simulink model "Simulation_wrapped_4"  (R2015a)
settings: Solver=ode4  SolverMode=SingleTasking  StartTime=0.0  StopTime=20  FixedStep=0.001  MaxStep=0.01  RelTol=1e-3
InitFcn:
  | gen_signal
  | Read_aero_spreadsheet
  | model_params3
undefined symbols (not defined in the file or in its folder): acm_aero_model, acm_pitch_deg_ini, acm_pitch_rate_deg_s_ini, acm_T_N, breakpoints1, Cm0, Cmde, Cmq, dail, de, dele, drud, Fr_mp_1, Fr_mp_2, Fr_rp_1, Fr_rp_2, ini_acm_de_deg, ini_acm_p_deg_per_s, ini_acm_phi_deg, ini_acm_psi_deg, ini_acm_q_deg_per_s, ini_acm_r_deg_per_s, ini_acm_theta_deg, ini_cmp_de_deg, ini_rig_p_deg_per_s, ini_rig_phi_deg, ini_rig_psi_deg, ini_rig_q_deg_per_s, ini_rig_r_deg_per_s, ini_rig_theta_deg, ini_rig_theta_deg_per_s, K1_svo_acm, K1_svo_cmp, K2_svo_acm, K2_svo_cmp, K_de_nz2, K_de_q2, K_de_tht2, La, Ma, max_defl_sat_acm, max_defl_sat_cmp, max_rate_sat, max_rate_sat_acm, max_rate_sat_cmp, Na, rig_pitch_deg_ini, rig_pitch_rate_deg_s_ini, sigbuilder_block, simstop, windspeed, Xa, Ya, Za
libraries: aerolibconvert2 x96, simulink x40, aerolibtransform2 x18, vrlib x7
(part 2 of 6)

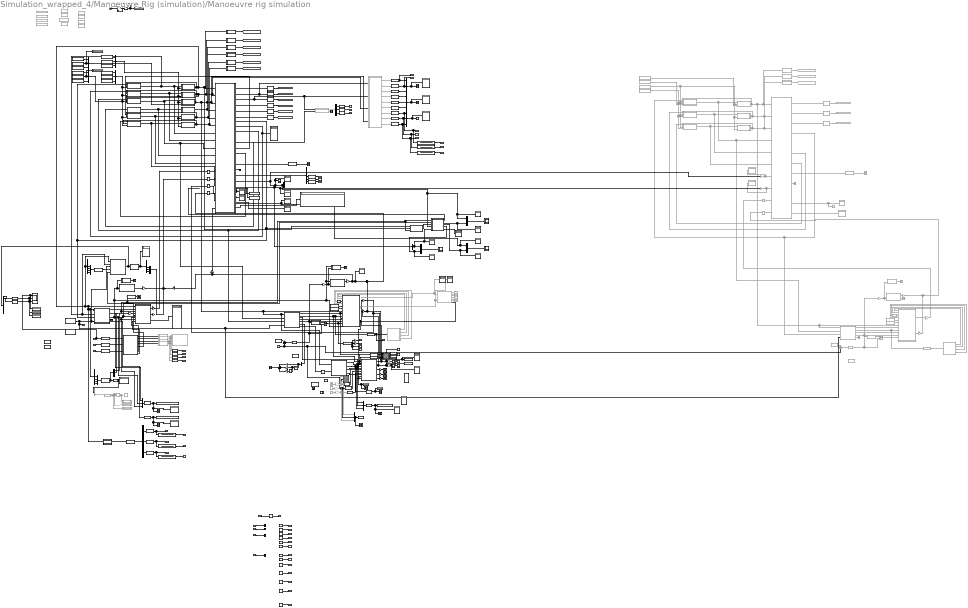
== system Simulation_wrapped_4/Manoeuvre Rig (simulation)/Manoeuvre rig simulation ==
  note: yaw
  note: pitch
  note: roll
  note: Estimated reaction forces
  note: Simulation aircraft reaction forces
  note: Estimated laod cell reading
  note: Simulation load cell reading
  note: ALTITUDE CONTROL
  note: Estimated estimated load cell moment
  note: Simulation load cell moment
  clock : Inport
  ACM_da_c(deg) : Inport  Port=2
  ACM_dea_c(deg) : Inport  Port=3
  ACM_de_c(deg) : Inport  Port=4
  ACM_dr_c(deg) : Inport  Port=5
  CMP_da_c(deg) : Inport  Port=6
  CMP_de_c(deg) : Inport  Port=7
  CMP_dr_c(deg) : Inport  Port=8
  extra : Inport  Port=9
  Aerodynamics lookup : Subsystem  Commented=on
  Aerodynamics lookup1 : Subsystem  Commented=on
  Aerodynamics model: Hawk : MATLAB Function
      settings: MinAlgLoopOccurrences=on
  Aerodynamics model: Hawk1 : MATLAB Function  Commented=on
      settings: MinAlgLoopOccurrences=on
  Aerodynamics model: compensator : MATLAB Function
      settings: MinAlgLoopOccurrences=on
  Aileron command (differential) : Terminator
  Aircraft acceleration body axis : MATLAB Function  Commented=on  TreatAsAtomicUnit=on
  Aircraft attitude relative to arm2 : MATLAB Function  Commented=on  TreatAsAtomicUnit=on
  Aircraft loads for load case loop : MATLAB Function  Commented=on
      settings: MinAlgLoopOccurrences=on
  Aircraft model vertical reaction force : Scope
      settings: YMin=5  YMax=24  SaveName=ScopeData38
  Aircraft model vertical reaction force1 : Scope  Commented=on
      settings: YMin=5  YMax=24
  Aircraft_model_friction : MATLAB Function
      settings: MinAlgLoopOccurrences=on
  Aircraft_model_friction1 : MATLAB Function  Commented=on
      settings: MinAlgLoopOccurrences=on
  Angle Conversion{,1,3,6,8..12,14..26,29..34,37..38,40} (31 alike) : aerolibconvert2/Angle Conversion  IU=rad  OU=deg
  Angle Conversion{2,4,7,13,27..28,35,39} (8 alike) : aerolibconvert2/Angle Conversion  IU=deg  OU=rad
  Angle Conversion36 : aerolibconvert2/Angle Conversion  Commented=on  IU=deg  OU=rad
  Angle Conversion44 : aerolibconvert2/Angle Conversion  Commented=on  IU=deg  OU=rad
  Angle Conversion5 : aerolibconvert2/Angle Conversion  Commented=on  IU=rad  OU=deg
  Angle of sideslip : Constant  Value=0
  Butterworth filter (cutoff frequency 10Hz) + differentiating{,1..5} (6 alike) : TransferFcn  Numerator=[1 0]  Denominator=[2.5330e-04 0.0225 1]
  CMP aero model : MATLABFcn  MATLABFcn=Cmp_aero_model
  Calculating rig pitch acceleration : MATLAB Function  TreatAsAtomicUnit=on
  Chirp Signal : simulink/Sources/Chirp Signal  Commented=on  f1=0.5  T=120  f2=3
  Chirp Signal1 : simulink/Sources/Chirp Signal  Commented=on  f1=0.5  T=120  f2=3
  Chirp Signal2 : simulink/Sources/Chirp Signal  f1=0.5  T=120  f2=3
  Clock : Clock
  Comparing simulation aircraft reaction forces and estimated reaction forces : Scope
      settings: YMin=-35  YMax=15  SaveName=ScopeData3
  Comparing simulation aircraft reaction forces and estimated reaction forces1 : Scope
      settings: YMin=-35  YMax=15  SaveName=ScopeData4
  Comparing simulation load cell reading and estimated load cell reading : Scope
      settings: YMin=-17.5  YMax=37.5  SaveName=ScopeData2
  Compensator friction : MATLAB Function
      settings: MinAlgLoopOccurrences=on
  Compensator servo model1 : Subsystem  Commented=on
  Compensator servo model2 : Subsystem  Commented=on
  Compensator servo model3 : Subsystem  Commented=on
  Compensator servo model4 : Subsystem  Commented=on
  Constant : Constant  Commented=on  Value=simstop
  Constant{1,7..8,12..13,19} (6 alike) : Constant  Commented=on  Value=0
  Constant10 : Constant  Value=7.515637662
  Constant11 : Constant  Value=0
  Constant14 : Constant  Commented=on  Value=2.6111
  Constant15 : Constant  Commented=on  Value=rig_pitch_rate_deg_s_ini
  Constant16 : Constant  Commented=on  Value=acm_pitch_rate_deg_s_ini
  Constant17 : Constant  Commented=on  Value=rig_pitch_deg_ini
  Constant18 : Constant  Commented=on  Value=acm_pitch_deg_ini
  Constant2 : Constant  Value=-7.308232274
  Constant3 : Constant  Value=14.34612797
  Constant4 : Constant  Commented=on  Value=-7.308232274
  Constant6 : Constant  Commented=on  Value=5
  Cq_transpose_lc CHECK : Display
  Demux : Demux  Outputs=7
  Demux{1..3,5..6,12} (6 alike) : Demux  Outputs=3
  Demux10 : Demux  Outputs=11
  Demux4 : Demux  Commented=on  Outputs=3
  Demux7 : Demux  Outputs=6
  Demux8 : Demux  Outputs=7
  Demux9 : Demux  Outputs=6
  Derivative : Derivative
  Display{,2..3,5..14,18} (14 alike) : Display
  Display{1,4,15..17} (5 alike) : Display  Commented=on
  Elevator command (differential) : Terminator
  Equations of Motion : MATLAB Function
      settings: MinAlgLoopOccurrences=on
  Equations of Motion1 : MATLAB Function  Commented=on
      settings: MinAlgLoopOccurrences=on
  Extra : Terminator
  Extracting aircraft vertical reaction forces1 : MATLAB Function  TreatAsAtomicUnit=on
  Extracting aircraft vertical reaction forces2 : MATLAB Function  Commented=on  TreatAsAtomicUnit=on
  Extracting position vector 1 : Subsystem
  Extracting position vector 10 : Subsystem  Commented=on
  Extracting position vector 2 : Subsystem
  "Extracting position vector 2 " : Subsystem
  Extracting position vector 3 : Subsystem
  Extracting position vector 4 : Subsystem
  Extracting position vector 5 : Subsystem
  Extracting position vector 7 : Subsystem  Commented=on
  Extracting position vector 8 : Subsystem  Commented=on
  F : Display
  FF : Display
  Fcn : Fcn  Expr=u/9.81
  Fcn1 : Fcn  Expr=u/9.81
  Fcn2 : Fcn  Expr=u/9.81
  Friction_estimate : Display
  Friction_moment : Display
  Gain{,3,6..7,11,14,28} (7 alike) : Gain  Gain=-1
  Gain1 : Gain  Commented=on  Gain=-1
  Gain{4,8..10,17,19..23,30} (11 alike) : Gain
  Gain12 : Gain  Gain=0
  Gain13 : Gain  Gain=0
  Gain15 : Gain  Commented=on  Gain=-1
  Gain16 : Gain  Commented=on  Gain=0
  Gain18 : Gain  Commented=on
  Gain2 : Gain  Commented=on
  Gain24 : Gain  Commented=on  Gain=dail
  Gain25 : Gain  Commented=on  Gain=dele
  Gain26 : Gain  Commented=on
  Gain27 : Gain  Commented=on  Gain=drud
  Goto10 : Goto  Commented=on  GotoTag=animation_l2_translation  TagVisibility=global
  Goto15 : Goto  Commented=on  GotoTag=animation_acm2_rotation  TagVisibility=global
  Goto16 : Goto  Commented=on  GotoTag=animation_lc2_rotation  TagVisibility=global
  Goto17 : Goto  Commented=on  GotoTag=animation_l2_rotation  TagVisibility=global
  Goto8 : Goto  Commented=on  GotoTag=animation_acm2_translation  TagVisibility=global
  Goto9 : Goto  Commented=on  GotoTag=animation_lc2_translation  TagVisibility=global
  HHIRM : MATLAB Function
      settings: MinAlgLoopOccurrences=on
  Hawk servo model : Subsystem
  Hawk servo model1 : Subsystem  Commented=on
  IC{1..4} (4 alike) : InitialCondition  Value=0
  IC7 : InitialCondition  Commented=on  Value=0
  IC8 : InitialCondition  Commented=on  Value=0
  Integrator : Integrator
  Integrator1 : Integrator
  L : Constant  Commented=on  Value=La
  Left aileron command : Constant  Value=0
  Left aileron measured : Constant  Value=0
  Load cell reading to aircraft reaction forces : MATLAB Function  TreatAsAtomicUnit=on
  M : Display
  M1 : Constant  Commented=on  Value=Ma
  MATLAB Function1 : MATLAB Function  TreatAsAtomicUnit=on
  MATLAB Function10 : MATLAB Function  TreatAsAtomicUnit=on
  MATLAB Function11 : MATLAB Function  Commented=on  TreatAsAtomicUnit=on
  MATLAB Function13 : MATLAB Function  Commented=on
      settings: MinAlgLoopOccurrences=on
  MATLAB Function15 : MATLAB Function  Commented=on  TreatAsAtomicUnit=on
  MATLAB Function18 : MATLAB Function  Commented=on  TreatAsAtomicUnit=on
  MATLAB Function2 : MATLAB Function  TreatAsAtomicUnit=on
  MATLAB Function3 : MATLAB Function
      settings: MinAlgLoopOccurrences=on
  MATLAB Function4 : MATLAB Function  TreatAsAtomicUnit=on
  MATLAB Function5 : MATLAB Function
      settings: MinAlgLoopOccurrences=on
  MATLAB Function6 : MATLAB Function  TreatAsAtomicUnit=on
  MATLAB Function7 : MATLAB Function
      settings: MinAlgLoopOccurrences=on
  MATLAB Function8 : MATLAB Function  TreatAsAtomicUnit=on
  MATLAB Function9 : MATLAB Function  TreatAsAtomicUnit=on
  MM : Display
  Manual Switch1 : ManualSwitch  CurrentSetting=0
  Manual Switch3 : ManualSwitch  Commented=on  CurrentSetting=0
  Memory : Memory
  Mux{,2..4,7..10,12..13,15} (11 alike) : Mux  Inputs=3
  Mux1 : Mux  Inputs=2
  Mux11 : Mux
  Mux14 : Mux
  Mux5 : Mux  Inputs=2
  Mux6 : Mux  Inputs=2
  N : Constant  Commented=on  Value=Na
  Physical deflections to virtual compensator deflections : MATLAB Function  Commented=on  TreatAsAtomicUnit=on
  Quaternions to Rotation Angles : aerolibtransform2/Quaternions to Rotation Angles  rotationOrder=ZYX
  Quaternions to Rotation Angles1 : aerolibtransform2/Quaternions to Rotation Angles  rotationOrder=ZYX
  Quaternions to Rotation Angles2 : aerolibtransform2/Quaternions to Rotation Angles  rotationOrder=ZYX
  Relational Operator : RelationalOperator  Commented=on  OutDataTypeStr=boolean
  Relative angle from rotation matrix : Scope
      settings: ShowLegends=on  YMax=12.5  SaveName=ScopeData17
  Right aileron command : Constant  Value=0
  Right aileron measured : Constant  Value=0
  Rotation angles from rotation matrix (acm) : Scope
      settings: ShowLegends=on  YMax=12.5  SaveName=ScopeData19
  Rotation angles from rotation matrix (arm) : Scope
      settings: ShowLegends=on  YMax=12.5  SaveName=ScopeData20
  Rudder command : Terminator
  Rudder measured : Constant  Value=0
  Rudder measured command : Constant  Value=0
  Scope{,1..8,10..13} (13 alike) : Scope
      Scope settings: YMin=-0.5  YMax=0.2  SaveName=ScopeData6
      Scope1 settings: YMin=0.12  YMax=0.1775  SaveName=ScopeData8
      Scope10 settings: YMin=-3.25  YMax=0  SaveName=ScopeData21
      Scope11 settings: YMin=-17.5  YMax=0  SaveName=ScopeData30
      Scope12 settings: YMin=0  YMax=1000  SaveName=ScopeData33
      Scope13 settings: YMin=-275  YMax=275  SaveName=ScopeData34
      Scope2 settings: YMin=0  YMax=14  SaveName=ScopeData9
      Scope3 settings: YMin=-700  YMax=700  SaveName=ScopeData10
      Scope4 settings: YMin=-8  YMax=8  SaveName=ScopeData11
      Scope5 settings: YMin=-21  YMax=1  SaveName=ScopeData12
      Scope6 settings: YMin=0  YMax=14  SaveName=ScopeData13
      Scope7 settings: YMin=0  YMax=14  SaveName=ScopeData15
      Scope8 settings: YMin=-0.02  YMax=0.0225  SaveName=ScopeData18
  Scope14 : Scope  NumInputPorts=3
      settings: YMin=38~127.5~-1240  YMax=42~157.5~-1190  SaveName=ScopeData35
  Scope9 : TimeScope  NumInputPorts=5
  Signal Builder : Subsystem  Tag=STV Subsys  LoadFcn=sigbuilder_block('load');  StartFcn=sigbuilder_block('start');  StopFcn=sigbuilder_block('stop');  ClipboardFcn=sigbuilder_block('clipboard');  mask(Sigbuilder block){}
      mask help: Simulink:masks:SigbuilderBlock_MD
      mask init:
      | if ~strcmp(get_param(bdroot(gcbh),'SimulationStatus'),'stopped') tuvar = sigbuilder_block('maskInit'); end
      settings: CopyFcn=sigbuilder_block('copy');  DeleteFcn=sigbuilder_block('delete');  ModelCloseFcn=sigbuilder_block('modelClose');  PreSaveFcn=sigbuilder_block('preSave');  PauseFcn=sigbuilder_block('pause');  ContinueFcn=sigbuilder_block('continue');  NameChangeFcn=sigbuilder_block('namechange');  OpenFcn=sigbuilder_block('open',[437.6 199.2 550.4 400 ]);  CloseFcn=sigbuilder_block('close');
      mask Display: plot(0, 0, 100, 100,[2, 2, 32, 32, 2], [68, 8, 8, 68, 68],[32, 2], [38, 38], [32, 19, 2],[53, 60, 44], [32, 17, 17, 2],[16, 16, 31, 31]);txt = getActiveGroup(gcbh);text(2, 100, txt,'verticalAlignment', 'top');
  Step : Step  Commented=on  Time=0.01  SampleTime=0
  Step2 : Step  SampleTime=0
  Step3 : Step  SampleTime=0
  Stop Simulation : Stop  Commented=on
  Subsystem : Subsystem
  Subsystem1 : Subsystem
  Subsystem10 : Subsystem
  Subsystem11 : Subsystem
  Subsystem12 : Subsystem
  Subsystem13 : Subsystem
  Subsystem16 : Subsystem  Commented=on
  Subsystem17 : Subsystem  Commented=on
  Subsystem18 : Subsystem  Commented=on
  Subsystem19 : Subsystem  Commented=on
  Subsystem2 : Subsystem
  Subsystem22 : Subsystem  Commented=on
  Subsystem23 : Subsystem  Commented=on
  Subsystem24 : Subsystem  Commented=on
  Subsystem3 : Subsystem
  Subsystem4 : Subsystem
  Subsystem5 : Subsystem
  Subsystem6 : Subsystem
  Subsystem7 : Subsystem
  Subsystem8 : Subsystem
  Subsystem9 : Subsystem
  Sum1 : Sum  Commented=on  Inputs=|++
  Sum2 : Sum  Inputs=|++
  Sum3 : Sum
  Sum4 : Sum  Commented=on
  Sum5 : Sum  Inputs=+++
  Sum8 : Sum  Inputs=++-
  Switch : Switch  Criteria=u2 > Threshold
  Terminator{,1..5} (6 alike) : Terminator
  Terminator{7..10} (4 alike) : Terminator  Commented=on
  Theta1 : Constant  Commented=on  Value=2.9881840554008
  To Workspace : ToWorkspace  VariableName=reaction_forces_lc_body_N  SaveFormat=Timeseries  SampleTime=-1
  To Workspace1 : ToWorkspace  VariableName=reaction_moments_lc_body_Nm  SaveFormat=Timeseries  SampleTime=-1
  To Workspace2 : ToWorkspace  VariableName=cs_deg  SaveFormat=Timeseries  SampleTime=-1
  To Workspace3 : ToWorkspace  VariableName=alpha_deg  SaveFormat=Timeseries  SampleTime=-1
  To Workspace4 : ToWorkspace  VariableName=beta_deg  SaveFormat=Timeseries  SampleTime=-1
  To Workspace5 : ToWorkspace  VariableName=aero_forces_N  SaveFormat=Timeseries  SampleTime=-1
  To Workspace6 : ToWorkspace  VariableName=aero_moments_Nm  SaveFormat=Timeseries  SampleTime=-1
  To Workspace7 : ToWorkspace  VariableName=wind_axes_rotation_rates_degpers  SaveFormat=Timeseries  SampleTime=-1
  To Workspace8 : ToWorkspace  VariableName=inertial_axes_CMP_rotation_rates_degpers  SaveFormat=Timeseries  SampleTime=-1
  To Workspace9 : ToWorkspace  VariableName=inertial_axes_CMP_rotation_accelerations_degperspers  SaveFormat=Timeseries  SampleTime=-1
  Transport Delay : TransportDelay  DelayTime=0.01
  Unused{,1..2,4,6,8} (6 alike) : Constant  Value=0
  V{,1..3} (4 alike) : Display
  Virtual compensator deflections to physical deflections : MATLAB Function  TreatAsAtomicUnit=on
  Wind axes angular rates calculation : MATLAB Function
      settings: MinAlgLoopOccurrences=on
  Wind tunnel velocity : Constant  Value=windspeed
  Wind tunnel velocity1 : Constant  Value=25.09344509
  X : Constant  Commented=on  Value=Xa
  Y : Constant  Commented=on  Value=Ya
  Z : Constant  Commented=on  Value=Za
  acm_T_N : Constant  Value=acm_T_N
  acm_T_N1 : Constant  Commented=on  Value=acm_T_N
  acm_aero_model : Constant  Value=acm_aero_model
  acm_aero_model1 : Constant  Commented=on  Value=acm_aero_model
  aircraft_cell_reaction_forces : Display
  aircraft_cell_reaction_moments : Display
  alpha : Display
  alpha1 : Display
  alpha2 : Scope
      settings: YMin=-55  YMax=55  SaveName=ScopeData22
  beta2 : Scope
      settings: YMin=-12.25  YMax=-8.75  SaveName=ScopeData23
  ini_acm_q_deg_per_s : Constant  Value=ini_acm_q_deg_per_s
  ini_acm_q_deg_per_s1 : Constant  Commented=on  Value=ini_acm_q_deg_per_s
  ini_acm_q_deg_per_s2 : Constant  Value=ini_acm_p_deg_per_s
  ini_acm_q_deg_per_s3 : Constant  Value=ini_acm_r_deg_per_s
  ini_acm_theta_deg : Constant  Value=ini_acm_theta_deg
  ini_acm_theta_deg1 : Constant  Commented=on  Value=ini_acm_theta_deg
  ini_acm_theta_deg2 : Constant  Value=ini_acm_phi_deg
  ini_acm_theta_deg3 : Constant  Value=ini_acm_psi_deg
  ini_rig_theta_deg : Constant  Value=ini_rig_theta_deg
  ini_rig_theta_deg1 : Constant  Commented=on  Value=ini_rig_theta_deg
  ini_rig_theta_deg2 : Constant  Value=ini_rig_psi_deg
  ini_rig_theta_deg3 : Constant  Value=ini_rig_phi_deg
  ini_rig_theta_deg_per_s : Constant  Value=ini_rig_q_deg_per_s
  ini_rig_theta_deg_per_s1 : Constant  Commented=on  Value=ini_rig_theta_deg_per_s
  ini_rig_theta_deg_per_s2 : Constant  Value=ini_rig_p_deg_per_s
  ini_rig_theta_deg_per_s3 : Constant  Value=ini_rig_r_deg_per_s
  load_cell_reaction_forces{,2..8} (8 alike) : Display
  load_cell_reaction_forces1 : Display  Commented=on
  load_cell_reaction_forces_body : Display
  load_cell_reaction_moments : Display
  load_cell_reaction_moments1 : Display  Commented=on
  load_cell_reaction_moments_body : Display
  q : Display
  q1 : Display
  rates : Display
  theta_rig : Scope
      settings: YMin=-29  YMax=-24.5  SaveName=ScopeData26
  z_reaction_force : Scope
      settings: YMin=-125  YMax=150  SaveName=ScopeData32
  z_reaction_force1 : Scope  Commented=on
      settings: YMax=70  SaveName=ScopeData5
  ACM_CmdTime : Outport
  GX(deg/s) : Outport  Port=2
  GY(deg/s) : Outport  Port=3
  GZ(deg/s) : Outport  Port=4
  Nx : Outport  Port=5
  Ny : Outport  Port=6
  Nz : Outport  Port=7
  ACM_roll(deg) : Outport  Port=8
  ACM_rollrate(deg/s) : Outport  Port=9
  ACM_pitch(deg) : Outport  Port=10
  ACM_pitchrate(deg/s) : Outport  Port=11
  ACM_yaw(deg) : Outport  Port=12
  ACM_yawrate(deg/s) : Outport  Port=13
  RIG_roll(deg) : Outport  Port=14
  RIG_rollrate(deg/s) : Outport  Port=15
  RIG_pitch(deg) : Outport  Port=16
  RIG_pitchrate(deg/s) : Outport  Port=17
  RIG_yaw(deg) : Outport  Port=18
  RIG_yawrate(deg/s) : Outport  Port=19
  delta_al_c(deg) : Outport  Port=20
  delta_al(deg) : Outport  Port=21
  delta_ar_c(deg) : Outport  Port=22
  delta_ar(deg) : Outport  Port=23
  delta_r_c(deg) : Outport  Port=24
  delta_r(deg) : Outport  Port=25
  delta_c(deg) : Outport  Port=26
  delta(deg) : Outport  Port=27
  delta_el_c(deg) : Outport  Port=28
  delta_el(deg) : Outport  Port=29
  delta_er_c(deg) : Outport  Port=30
  delta_er(deg) : Outport  Port=31
  delta_cmp1_c(deg) : Outport  Port=32
  delta_cmp1(deg) : Outport  Port=33
  delta_cmp2_c(deg) : Outport  Port=34
  delta_cmp2(deg) : Outport  Port=35
  delta_cmp3_c(deg) : Outport  Port=36
  delta_cmp3(deg) : Outport  Port=37
  delta_cmp4_c(deg) : Outport  Port=38
  delta_cmp4(deg) : Outport  Port=39
  wind speed(m/s) : Outport  Port=40
  AoA(deg) : Outport  Port=41
  AoS(deg) : Outport  Port=42
  roll_ac(deg) : Outport  Port=43
  pitch_ac(deg) : Outport  Port=44
  tag scope: animation_acm_rotation=global, animation_acm_translation=global, animation_arm_rotation=global, animation_arm_translation=global, animation_cmp_rotation=global, animation_cmp_translation=global, animation_link_rotation=global, animation_link_translation=global, animation_load_cell_rotation=global, animation_load_cell_translation=global, animation_mass_rotation=global, animation_mass_translation=global
  wires:
  Equations of Motion/2(Ar) -> Aircraft attitude relative to arm2/1(Ar), MATLAB Function1/1(A2)
  Equations of Motion/8(qr_dot_dot) -> Subsystem2/1(In1), load_cell_reaction_forces8/1
  Subsystem2/1(Out1) -> Equations of Motion/8(qr_dot), Subsystem3/1(In1)
  Angle Conversion2/1 -> Hawk servo model/1(Command), Manual Switch1/2
  Sum3/1 -> Angle Conversion2/1  "Hawk elevator (deg)"
  Equations of Motion/11(qm_dot_dot) -> Subsystem8/1(In1)
  Subsystem8/1(Out1) -> Equations of Motion/10(qm_dot), Subsystem9/1(In1)
  Subsystem9/1(Out1) -> Extracting position vector 4/1(In1), Equations of Motion/4(qm)
  Equations of Motion/4(Am) -> MATLAB Function8/1(A3)
  Compensator friction/1(Fr_rp) -> Gain12/1
  Extracting aircraft vertical reaction forces1/1(RF_a) -> Aircraft model vertical reaction force/1
  Gain13/1 -> Friction_moment/1, Sum2/1, Gain30/1, Gain3/1  "Friction moment"
  Gain30/1 -> Sum8/3
  Gain20/1 -> Subsystem6/2(theta_dot_mp), Aircraft_model_friction/2(theta_dot_mp)
  Equations of Motion/14(RF) -> Extracting aircraft vertical reaction forces1/1(RF)
  Angle Conversion1/1 -> AoA(deg)/1, Aerodynamics lookup/1(Alpha (deg))  "Hawk alpha (deg)"
  MATLAB Function4/1(q2) -> Quaternions to Rotation Angles/1
  Quaternions to Rotation Angles/1 -> Demux3/1
  Demux3/2 -> Angle Conversion9/1
  Aircraft acceleration body axis/1(qa_dot_dot3) -> Demux5/1
  Integrator/1 -> Integrator1/1, Gain/1
  Demux6/3 -> Gain7/1, Integrator/1
  Gain/1 -> Sum5/2
  Integrator1/1 -> Gain6/1
  Gain6/1 -> Sum5/3
  Gain7/1 -> Sum5/1
  Demux3/1 -> Angle Conversion8/1
  Butterworth filter (cutoff frequency 10Hz) + differentiating/1 -> RIG_rollrate(deg/s)/1
  Butterworth filter (cutoff frequency 10Hz) + differentiating2/1 -> RIG_yawrate(deg/s)/1
  Demux3/3 -> Angle Conversion10/1
  Angle Conversion8/1 -> RIG_roll(deg)/1, Butterworth filter (cutoff frequency 10Hz) + differentiating/1
  Angle Conversion9/1 -> Butterworth filter (cutoff frequency 10Hz) + differentiating1/1, RIG_pitch(deg)/1
  Angle Conversion10/1 -> RIG_yaw(deg)/1, Butterworth filter (cutoff frequency 10Hz) + differentiating2/1
  Demux5/1 -> Fcn/1
  Demux5/2 -> Fcn1/1
  Demux5/3 -> Fcn2/1
  Equations of Motion/16(qa_dot2) -> Demux7/1
  Demux7/4 -> Angle Conversion/1
  Demux7/5 -> Angle Conversion11/1
  Demux7/6 -> Angle Conversion12/1
  Fcn/1 -> Nx/1
  Fcn1/1 -> Ny/1
  Fcn2/1 -> Nz/1
  Angle Conversion/1 -> GX(deg/s)/1
  Angle Conversion11/1 -> GY(deg/s)/1
  Angle Conversion12/1 -> GZ(deg/s)/1
  Subsystem3/1(Out1) -> Subsystem2/2(q), Subsystem4/5(qr), "Extracting position vector 2 "/1(In1), Equations of Motion/2(qr), Aircraft attitude relative to arm2/3(qr)
  Equations of Motion/3(Aa) -> MATLAB Function6/1(A3), Aircraft acceleration body axis/1(Aa), Aircraft attitude relative to arm2/2(Aa)
  Mux2/1 -> Relative angle from rotation matrix/1, Display/1
  Aircraft attitude relative to arm2/7(phi_relative) -> Angle Conversion16/1
  Aircraft attitude relative to arm2/9(psi_relative) -> Angle Conversion18/1
  Angle Conversion18/1 -> Butterworth filter (cutoff frequency 10Hz) + differentiating5/1, ACM_yaw(deg)/1, Mux2/3  "Yaw"
  Angle Conversion17/1 -> Mux2/2, Butterworth filter (cutoff frequency 10Hz) + differentiating4/1, ACM_pitch(deg)/1  "Pitch"
  Angle Conversion16/1 -> ACM_roll(deg)/1, Butterworth filter (cutoff frequency 10Hz) + differentiating3/1, Mux2/1  "Roll"
  Mux3/1 -> Display2/1, Rotation angles from rotation matrix (acm)/1
  Angle Conversion21/1 -> Mux3/3  "Yaw"
  Angle Conversion20/1 -> pitch_ac(deg)/1, Mux3/2  "Pitch"
  Angle Conversion19/1 -> roll_ac(deg)/1, Mux3/1  "Roll"
  Aircraft attitude relative to arm2/1(phi_acm) -> Angle Conversion19/1
  Aircraft attitude relative to arm2/2(theta_acm) -> Angle Conversion20/1
  Aircraft attitude relative to arm2/3(psi_acm) -> Angle Conversion21/1
  Mux4/1 -> Rotation angles from rotation matrix (arm)/1, Display3/1
  Angle Conversion24/1 -> Mux4/3  "Yaw"
  Angle Conversion23/1 -> Mux4/2  "Pitch"
  Angle Conversion22/1 -> Mux4/1  "Roll"
  Aircraft attitude relative to arm2/4(phi_arm) -> Angle Conversion22/1
  Aircraft attitude relative to arm2/5(theta_arm) -> Angle Conversion23/1
  Aircraft attitude relative to arm2/6(psi_arm) -> Angle Conversion24/1
  clock/1 -> Transport Delay/1
  Transport Delay/1 -> ACM_CmdTime/1
  Butterworth filter (cutoff frequency 10Hz) + differentiating3/1 -> ACM_rollrate(deg/s)/1
  Butterworth filter (cutoff frequency 10Hz) + differentiating4/1 -> ACM_pitchrate(deg/s)/1
  Butterworth filter (cutoff frequency 10Hz) + differentiating5/1 -> ACM_yawrate(deg/s)/1
  Left aileron command/1 -> delta_al_c(deg)/1
  Left aileron measured/1 -> delta_al(deg)/1
  Right aileron command/1 -> delta_ar_c(deg)/1
  Right aileron measured/1 -> delta_ar(deg)/1
  Rudder measured command/1 -> delta_r_c(deg)/1
  Rudder measured/1 -> delta_r(deg)/1
  Unused/1 -> delta_c(deg)/1
  Unused1/1 -> delta(deg)/1
  Unused2/1 -> delta_cmp1_c(deg)/1
  Unused4/1 -> delta_cmp2_c(deg)/1
  Unused6/1 -> delta_cmp3_c(deg)/1
  Unused8/1 -> delta_cmp4_c(deg)/1
  Angle of sideslip/1 -> AoS(deg)/1
  ACM_da_c(deg)/1 -> Aileron command (differential)/1
  ACM_dea_c(deg)/1 -> Elevator command (differential)/1
  ACM_dr_c(deg)/1 -> Rudder command/1
  CMP_da_c(deg)/1 -> Display12/1, Scope14/1, Angle Conversion35/1  "input (deg)"
  CMP_dr_c(deg)/1 -> Angle Conversion39/1
  extra/1 -> Extra/1
  Angle Conversion6/1 -> Gain11/1, Gain14/1, delta_er(deg)/1, delta_er_c(deg)/1
  Virtual compensator deflections to physical deflections/1(servo1) -> Compensator servo model1/1(Command)
  Virtual compensator deflections to physical deflections/2(servo2) -> Compensator servo model2/1(Command)
  Virtual compensator deflections to physical deflections/3(servo3) -> Compensator servo model3/1(Command)
  Virtual compensator deflections to physical deflections/4(servo4) -> Compensator servo model4/1(Command)
  Angle Conversion4/1 -> Aerodynamics model: Hawk/3(de)
  Aerodynamics lookup/1(Cm0) -> Aerodynamics model: Hawk/1(Cm0)
  Aerodynamics lookup/2(Cmde) -> Aerodynamics model: Hawk/2(Cmde)
  Aerodynamics lookup/3(de_deg) -> Angle Conversion4/1
  Aerodynamics lookup/4(Cmq) -> Aerodynamics model: Hawk/4(Cmq)
  Angle Conversion14/1 -> delta_cmp1(deg)/1
  Angle Conversion15/1 -> delta_cmp2(deg)/1
  Angle Conversion25/1 -> delta_cmp3(deg)/1
  Angle Conversion26/1 -> delta_cmp4(deg)/1
  MATLAB Function2/1(A11) -> [animation_cmp_rotation]
  MATLAB Function1/1(A22) -> [animation_arm_rotation]
  MATLAB Function6/1(A33) -> [animation_acm_rotation]
  MATLAB Function8/1(A33) -> [animation_mass_rotation]
  Extracting position vector 1/1(Out1) -> [animation_cmp_translation]
  "Extracting position vector 2 "/1(Out1) -> [animation_arm_translation]
  Extracting position vector 3/1(Out1) -> [animation_acm_translation]
  Extracting position vector 4/1(Out1) -> [animation_mass_translation]
  Compensator servo model1/1(Response) -> Angle Conversion14/1, Physical deflections to virtual compensator deflections/1(servo1)
  Compensator servo model2/1(Response) -> Angle Conversion15/1, Physical deflections to virtual compensator deflections/2(servo2)
  Compensator servo model3/1(Response) -> Angle Conversion25/1, Physical deflections to virtual compensator deflections/3(servo3)
  Compensator servo model4/1(Response) -> Angle Conversion26/1, Physical deflections to virtual compensator deflections/4(servo4)
  Equations of Motion/1(Ac) -> MATLAB Function2/1(A1)
  Manual Switch1/1 -> Angle Conversion6/1, Aerodynamics model: Hawk/12(eta)
  Virtual compensator deflections to physical deflections/7(de_cmp2) -> Aerodynamics model: compensator/6(eta)
  MATLAB Function7/1(V_t) -> Aerodynamics model: compensator/2(V_t)
  MATLAB Function3/1(V0) -> HHIRM/11(V), Scope6/1, V/1, Aerodynamics model: Hawk/8(V0)
  MATLAB Function3/2(alpha) -> Angle Conversion3/1, HHIRM/1(alpha), Angle Conversion1/1, Aerodynamics model: Hawk/9(alpha)
  MATLAB Function3/4(w_dot) -> Aerodynamics model: Hawk/10(w_dot)
  MATLAB Function3/5(q) -> Gain20/1, Aerodynamics model: Hawk/11(q)
  MATLAB Function3/6(Va) -> Demux6/1
  Aerodynamics model: compensator/1(F_c) -> Gain4/1
  Aerodynamics model: compensator/2(M_dash_c) -> Gain8/1
  Gain12/1 -> Sum8/1
  Equations of Motion/10(qa_dot_dot2) -> Aircraft acceleration body axis/2(qa_dot_dot2)
  Aircraft attitude relative to arm2/8(theta_relative) -> Angle Conversion17/1
  Aircraft_model_friction/1(Fr_mp) -> Gain13/1
  Mux15/1 -> Sum8/2
  Hawk servo model/1(Response) -> Manual Switch1/1
  Gain4/1 -> IC1/1
  Sum8/1 -> IC2/1
  Gain10/1 -> Scope5/1, IC3/1
  Sum2/1 -> IC4/1
  Subsystem5/1(Out1) -> Extracting position vector 3/1(In1), Equations of Motion/3(qa), Aircraft attitude relative to arm2/4(qa), Wind axes angular rates calculation/1(qa), MATLAB Function3/1(qa), Aerodynamics model: Hawk/7(qa), Subsystem4/2(qa)
  Subsystem4/1(Out1) -> Subsystem5/1(In1), MATLAB Function3/2(qa_dot), Equations of Motion/9(qa_dot)
  Equations of Motion/9(qa_dot_dot) -> Subsystem4/1(In1), MATLAB Function3/3(qa_dot_dot)
  IC1/1 -> Equations of Motion/13(F_c)
  IC2/1 -> Equations of Motion/14(M_dash_c)
  IC3/1 -> Equations of Motion/15(F_a)
  IC4/1 -> Equations of Motion/16(M_dash_a)
  Mux8/1 -> Subsystem1/2(rig attitude), Subsystem3/2(rig attitude), Subsystem5/2(rig attitude), Subsystem11/2(rig attitude), Subsystem13/2(rig attitude)
  Mux/1 -> Subsystem5/3(acm attitude)
  Switch/1 -> Memory/1
  Clock/1 -> Switch/2
  Memory/1 -> Display7/1, Switch/1
  Gain11/1 -> delta_el_c(deg)/1
  Gain14/1 -> delta_el(deg)/1
  Angle Conversion13/1 -> Virtual compensator deflections to physical deflections/2(de_cmp)
  CMP_de_c(deg)/1 -> Angle Conversion13/1  "Compensator elevator (deg)"
  Mux13/1 -> Subsystem4/3(rotation_rates), Subsystem12/3(rotation_rates), Subsystem10/3(rotation_rates), Subsystem2/3(rotation_rates), Subsystem/3(rotation_rates)
  Mux7/1 -> Subsystem4/4(angular rates (body))
  Subsystem10/1(Out1) -> Equations of Motion/11(qlc_dot), Subsystem11/1(In1)
  Equations of Motion/12(qlc_dot_dot) -> Subsystem10/1(In1)
  Subsystem13/1(Out1) -> Subsystem12/2(q), Equations of Motion/6(ql), Extracting position vector 5/1(In1)
  Equations of Motion/13(ql_dot_dot) -> Subsystem12/1(In1)
  Extracting position vector 2/1(Out1) -> [animation_load_cell_translation]
  Extracting position vector 5/1(Out1) -> [animation_link_translation]
  Subsystem11/1(Out1) -> Subsystem10/2(q), Extracting position vector 2/1(In1), Equations of Motion/5(qlc)
  MATLAB Function9/1(A33) -> [animation_load_cell_rotation]
  MATLAB Function10/1(A33) -> [animation_link_rotation]
  Equations of Motion/5(Alc) -> MATLAB Function9/1(A3)
  Equations of Motion/6(Al) -> MATLAB Function10/1(A3)
  Subsystem12/1(Out1) -> Equations of Motion/12(ql_dot), Subsystem13/1(In1)
  Aircraft acceleration body axis/2(nz) -> Terminator/1
  Equations of Motion/15(RF_arm) -> Terminator1/1
  MATLAB Function7/6(Vc) -> Terminator2/1
  Subsystem7/1(Fr_mp) -> Terminator3/1
  Subsystem6/1(Fr_mp) -> Terminator4/1
  Sum5/1 -> Terminator5/1  "de_acm"
  Constant11/1 -> Sum3/1
  acm_T_N/1 -> Aerodynamics model: Hawk/5(T)
  acm_aero_model/1 -> Aerodynamics model: Hawk/6(acm_aero_model)
  Butterworth filter (cutoff frequency 10Hz) + differentiating1/1 -> RIG_pitchrate(deg/s)/1
  Angle Conversion36/1 -> Hawk servo model1/1(Command), Manual Switch3/2
  Sum4/1 -> Angle Conversion36/1  "Hawk elevator (deg)"
  Extracting aircraft vertical reaction forces2/1(RF_a) -> Aircraft model vertical reaction force1/1
  Gain16/1 -> Sum1/1  "Friction moment"
  Gain18/1 -> Subsystem24/2(theta_dot_mp), Aircraft_model_friction1/2(theta_dot_mp)
  Equations of Motion1/8(RF) -> Extracting aircraft vertical reaction forces2/1(RF)
  Angle Conversion5/1 -> Aerodynamics lookup1/1(Alpha (deg))  "Hawk alpha (deg)"
  Equations of Motion1/1(Aa) -> MATLAB Function15/1(A3)
  Angle Conversion44/1 -> Aerodynamics model: Hawk1/3(de)
  Aerodynamics lookup1/1(Cm0) -> Aerodynamics model: Hawk1/1(Cm0)
  Aerodynamics lookup1/2(Cmde) -> Aerodynamics model: Hawk1/2(Cmde)
  Aerodynamics lookup1/3(de_deg) -> Angle Conversion44/1
  Aerodynamics lookup1/4(Cmq) -> Aerodynamics model: Hawk1/4(Cmq)
  Manual Switch3/1 -> Aerodynamics model: Hawk1/12(eta)
  MATLAB Function13/1(V0) -> Aerodynamics model: Hawk1/8(V0)
  MATLAB Function13/2(alpha) -> Angle Conversion5/1, Aerodynamics model: Hawk1/9(alpha)
  MATLAB Function13/3(w_dot) -> Aerodynamics model: Hawk1/10(w_dot)
  MATLAB Function13/4(q) -> Gain18/1, Aerodynamics model: Hawk1/11(q)
  Aerodynamics model: Hawk1/1(F_a) -> Gain2/1
  Aerodynamics model: Hawk1/2(M_dash_a) -> Gain26/1
  Aircraft_model_friction1/1(Fr_mp) -> Gain16/1
  Gain26/1 -> Sum1/2
  Hawk servo model1/1(Response) -> Manual Switch3/1
  Gain2/1 -> IC7/1
  Sum1/1 -> IC8/1
  Subsystem23/1(Out1) -> Subsystem22/2(q), MATLAB Function13/1(qa), Aerodynamics model: Hawk1/7(qa), Equations of Motion1/1(qa), Extracting position vector 8/1(In1)
  Subsystem22/1(Out1) -> Subsystem23/1(In1), MATLAB Function13/2(qa_dot), Equations of Motion1/4(qa_dot)
  Equations of Motion1/4(qa_dot_dot) -> Subsystem22/1(In1), MATLAB Function13/3(qa_dot_dot)
  IC7/1 -> Equations of Motion1/9(F_a)
  IC8/1 -> Equations of Motion1/10(M_dash_a)
  ini_rig_theta_deg1/1 -> Subsystem18/3(theta_rig), Subsystem16/3(theta_rig), Subsystem22/3(theta_rig), Subsystem19/2(theta_rig), Subsystem17/2(theta_rig), Subsystem23/2(theta_rig)
  ini_acm_theta_deg1/1 -> Subsystem23/3(pitch_acm_ini)
  ini_rig_theta_deg_per_s1/1 -> Subsystem18/4(q_rig), Subsystem16/4(q_rig), Subsystem22/4(q_rig)
  ini_acm_q_deg_per_s1/1 -> Subsystem22/5(q_acm)
  Subsystem16/1(Out1) -> Equations of Motion1/5(qlc_dot), Subsystem17/1(In1)
  Equations of Motion1/6(qlc_dot_dot) -> Subsystem16/1(In1)
  Subsystem19/1(Out1) -> Subsystem18/2(q), Equations of Motion1/3(ql), Extracting position vector 10/1(In1)
  Equations of Motion1/7(ql_dot_dot) -> Subsystem18/1(In1)
  Subsystem17/1(Out1) -> Subsystem16/2(q), Equations of Motion1/2(qlc), Extracting position vector 7/1(In1)
  Equations of Motion1/2(Alc) -> MATLAB Function18/1(A3)
  Equations of Motion1/3(Al) -> MATLAB Function11/1(A3)
  Subsystem18/1(Out1) -> Equations of Motion1/6(ql_dot), Subsystem19/1(In1)
  Equations of Motion1/12(reaction_moments) -> load_cell_reaction_moments1/1
  Equations of Motion1/11(reaction_forces) -> z_reaction_force1/1, load_cell_reaction_forces1/1
  Equations of Motion1/9(RF_arm) -> Terminator7/1
  Subsystem24/1(Fr_mp) -> Terminator10/1
  Constant1/1 -> Sum4/1
  acm_T_N1/1 -> Aerodynamics model: Hawk1/5(T)
  acm_aero_model1/1 -> Aerodynamics model: Hawk1/6(acm_aero_model)
  Aircraft_model_friction1/2(theta_dot_relative) -> Terminator8/1
  MATLAB Function13/5(Va) -> Terminator9/1
  Wind tunnel velocity/1 -> wind speed(m/s)/1, MATLAB Function13/4(Vt), MATLAB Function3/4(Vt), MATLAB Function5/3(Vt), MATLAB Function7/4(Vt)
  Equations of Motion/17(reaction_forces_lc) -> z_reaction_force/1, load_cell_reaction_forces/1, Load cell reading to aircraft reaction forces/4(R_reading), load_cell_reaction_forces2/1, Mux1/1, Demux12/1, Gain1/1
  Gain15/1 -> Display4/1, Equations of Motion1/8(M_dash_lc)
  Extracting position vector 8/1(Out1) -> Goto8/1
  Extracting position vector 7/1(Out1) -> Goto9/1
  Extracting position vector 10/1(Out1) -> Goto10/1
  MATLAB Function15/1(A33) -> Goto15/1
  MATLAB Function18/1(A33) -> Goto16/1
  MATLAB Function11/1(A33) -> Goto17/1
  Gain1/1 -> Display1/1, Equations of Motion1/7(F_lc)
  Equations of Motion/22(reaction_moments_a) -> aircraft_cell_reaction_moments/1
  Demux2/2 -> Angle Conversion31/1, Calculating rig pitch acceleration/3(theta_r), Load cell reading to aircraft reaction forces/1(theta_r), Aerodynamics model: compensator/3(alpha)
  Load cell reading to aircraft reaction forces/1(F_acm) -> ?
  Mux1/1 -> Comparing simulation load cell reading and estimated load cell reading/1
  Load cell reading to aircraft reaction forces/2(R) -> load_cell_reaction_forces3/1, Mux1/2
  Calculating rig pitch acceleration/1(theta_r_dot_dot) -> Load cell reading to aircraft reaction forces/3(theta_r_dot_dot)
  Mux5/1 -> Comparing simulation aircraft reaction forces and estimated reaction forces/1
  Load cell reading to aircraft reaction forces/3(R_a) -> load_cell_reaction_forces5/1, Mux5/2
  Equations of Motion/21(reaction_forces_a) -> aircraft_cell_reaction_forces/1, load_cell_reaction_forces4/1, Mux5/1
  Mux6/1 -> Comparing simulation aircraft reaction forces and estimated reaction forces1/1
  Load cell reading to aircraft reaction forces/4(M) -> load_cell_reaction_forces7/1, Mux6/2
  Equations of Motion/18(reaction_moments_lc) -> Demux1/1, load_cell_reaction_moments/1, Gain15/1
  Demux1/2 -> Mux6/1, Load cell reading to aircraft reaction forces/5(M_reading), load_cell_reaction_forces6/1
  Gain3/1 -> Equations of Motion/17(M_dash_l)
  Load cell reading to aircraft reaction forces/5(Friction_estimate) -> Friction_estimate/1
  MATLAB Function3/7(qa_wind) -> Derivative/1
  Derivative/1 -> Wind axes angular rates calculation/2(qa_wind_dot)
  Wind axes angular rates calculation/1(p) -> Mux10/1, HHIRM/3(p)
  Wind axes angular rates calculation/3(r) -> Mux10/3, HHIRM/5(r)
  MATLAB Function3/3(beta) -> Angle Conversion30/1, HHIRM/2(beta)
  Gain17/1 -> Scope/1
  HHIRM/5(CZ) -> Gain17/1
  Wind axes angular rates calculation/4(A_b2w) -> HHIRM/9(A_b2w)
  Gain19/1 -> Scope1/1
  HHIRM/3(CX) -> Gain19/1
  Gain21/1 -> Scope2/1
  HHIRM/4(CY) -> Gain21/1
  Gain22/1 -> Scope3/1
  Gain23/1 -> M/1, Scope4/1
  ini_acm_theta_deg3/1 -> Mux/1
  ini_acm_theta_deg/1 -> Display5/1, Mux/2
  ini_acm_theta_deg2/1 -> Mux/3
  ini_acm_q_deg_per_s2/1 -> Mux7/1
  ini_acm_q_deg_per_s3/1 -> Mux7/3
  ini_rig_theta_deg/1 -> Mux8/2
  ini_rig_theta_deg2/1 -> Mux8/1
  ini_rig_theta_deg3/1 -> Mux8/3
  Angle Conversion3/1 -> alpha2/1, To Workspace3/1, alpha/1
  Equations of Motion/19(reaction_forces_lc_body) -> To Workspace/1, load_cell_reaction_forces_body/1
  Equations of Motion/20(reaction_moments_lc_body) -> load_cell_reaction_moments_body/1, To Workspace1/1
  Step/1 -> Gain24/1
  Chirp Signal/1 -> Gain25/1
  Chirp Signal1/1 -> Gain27/1
  Gain24/1 -> V1/1, Mux9/1, Angle Conversion7/1
  ACM_de_c(deg)/1 -> Angle Conversion27/1, Mux9/2, V2/1, Sum4/2, Sum3/2
  Angle Conversion7/1 -> HHIRM/6(dail)
  Angle Conversion27/1 -> HHIRM/7(dele)
  Angle Conversion28/1 -> HHIRM/8(drud)
  Wind axes angular rates calculation/2(q) -> Angle Conversion29/1, Mux10/2, HHIRM/4(q)
  Angle Conversion29/1 -> q/1, Scope7/1
  Gain27/1 -> V3/1, Mux9/3, Angle Conversion28/1
  Gain9/1 -> Scope8/1, Sum2/2
  HHIRM/2(M_dash_a) -> Gain9/1, To Workspace6/1, Gain23/1
  HHIRM/1(Fa) -> Gain10/1, F/1, To Workspace5/1, Gain22/1
  Mux9/1 -> Scope10/1, To Workspace2/1
  Angle Conversion30/1 -> beta2/1, To Workspace4/1, alpha1/1
  Angle Conversion31/1 -> theta_rig/1
  Mux10/1 -> Angle Conversion32/1
  Angle Conversion32/1 -> To Workspace7/1, rates/1, Scope11/1
  Quaternions to Rotation Angles1/1 -> Demux2/1, Angle Conversion33/1
  Angle Conversion33/1 -> Demux4/1, Display6/1
  Demux/7 -> Mux11/4
  Demux/6 -> Mux11/3
  Demux/5 -> Mux11/2
  Demux/4 -> Mux11/1
  Mux11/1 -> Quaternions to Rotation Angles1/1
  MATLAB Function7/3(p) -> Mux12/1
  MATLAB Function7/5(r) -> Aerodynamics model: compensator/7(r), Mux12/3
  MATLAB Function7/4(q) -> Aerodynamics model: Hawk/13(q_rig), Subsystem6/1(theta_dot_rp), Aircraft_model_friction/1(theta_dot_rp), Subsystem7/1(theta_dot_rp), Compensator friction/1(theta_dot_rp), Mux12/2, Load cell reading to aircraft reaction forces/2(theta_r_dot), Aerodynamics model: compensator/5(q)
  Mux12/1 -> Angle Conversion34/1
  Equations of Motion/7(qc_dot_dot) -> Subsystem/1(In1), MATLAB Function7/3(qc_dot_dot), Calculating rig pitch acceleration/2(qc_dot_dot)
  Subsystem/1(Out1) -> MATLAB Function7/2(qc_dot), MATLAB Function5/2(qc_dot), Equations of Motion/7(qc_dot), Subsystem1/1(In1)
  Angle Conversion37/1 -> Scope13/1, Display11/1, To Workspace9/1
  MATLAB Function7/7(omega_dashc_dot) -> Angle Conversion37/1
  ini_rig_theta_deg_per_s/1 -> Mux13/2
  ini_rig_theta_deg_per_s3/1 -> Mux13/3
  ini_rig_theta_deg_per_s2/1 -> Mux13/1
  Angle Conversion35/1 -> Virtual compensator deflections to physical deflections/1(da_cmp)
  Angle Conversion39/1 -> Virtual compensator deflections to physical deflections/3(dr_cmp)
  ini_acm_q_deg_per_s/1 -> Display8/1, Mux7/2
  Angle Conversion34/1 -> To Workspace8/1, Display9/1, Scope12/1
  Constant/1 -> Display17/1, Relational Operator/2
  Demux8/7 -> Mux14/4
  Demux8/6 -> Mux14/3
  Demux8/5 -> Mux14/2
  Demux8/4 -> Mux14/1
  Mux14/1 -> Quaternions to Rotation Angles2/1
  Subsystem1/1(Out1) -> Subsystem/2(q), Calculating rig pitch acceleration/1(qc), Extracting position vector 1/1(In1), Equations of Motion/1(qc), Aerodynamics model: compensator/1(qc), MATLAB Function4/1(q1), Demux/1, MATLAB Function7/1(qc), MATLAB Function5/1(qc), Demux8/1
  Quaternions to Rotation Angles2/1 -> MATLAB Function5/4(rotation_angles)
  MATLAB Function5/1(input) -> Demux10/1, CMP aero model/1
  Virtual compensator deflections to physical deflections/5(s2) -> MATLAB Function5/5(s)
  CMP aero model/1 -> Demux9/1, Display10/1
  Demux9/6 -> Mux15/3
  Demux9/5 -> Mux15/2
  Demux9/4 -> Mux15/1
  Demux10/1 -> Angle Conversion38/1
  Demux10/2 -> Angle Conversion40/1
  Angle Conversion38/1 -> Display13/1, Scope14/2  "phi (deg)"
  Angle Conversion40/1 -> Display14/1, Scope14/3  "p (deg/s)"
  Relational Operator/1 -> Display15/1
  Demux4/3 -> Display16/1, Relational Operator/1
  Aerodynamics model: Hawk/3(Aa) -> Aircraft loads for load case loop/7(A_b2i), HHIRM/10(A_b2i)
  Aircraft loads for load case loop/1(Fa) -> FF/1
  X/1 -> Aircraft loads for load case loop/1(X)
  Y/1 -> Aircraft loads for load case loop/2(Y)
  Z/1 -> Aircraft loads for load case loop/3(Z)
  L/1 -> Aircraft loads for load case loop/4(L)
  M1/1 -> Aircraft loads for load case loop/5(M)
  N/1 -> Aircraft loads for load case loop/6(N)
  Aircraft loads for load case loop/2(M_dash_a) -> MM/1
  Equations of Motion/23(Cq_transpose_lc_reaction) -> Cq_transpose_lc CHECK/1
  Gain28/1 -> Aerodynamics model: compensator/4(beta)
  Demux2/1 -> Gain28/1
  Virtual compensator deflections to physical deflections/8(dr_cmp2) -> Aerodynamics model: compensator/8(rudd)
  Aerodynamics model: compensator/3(extra) -> Display18/1

== system Simulation_wrapped_4/Manoeuvre Rig (simulation)/Manoeuvre rig simulation/Aerodynamics lookup ==
  Alpha (deg) : Inport
  1-D Lookup Table : Lookup_n-D  NumberOfTableDimensions=1  BreakpointsForDimension1=breakpoints1  Table=de  DiagnosticForOutOfRangeInput=Warning  InternalRulePriority=Speed  RndMeth=Simplest  InputSameDT=on
  1-D Lookup Table1 : Lookup_n-D  NumberOfTableDimensions=1  BreakpointsForDimension1=breakpoints1  Table=Cm0  DiagnosticForOutOfRangeInput=Warning  InternalRulePriority=Speed  RndMeth=Simplest  InputSameDT=on
  1-D Lookup Table2 : Lookup_n-D  NumberOfTableDimensions=1  BreakpointsForDimension1=breakpoints1  Table=Cmde  DiagnosticForOutOfRangeInput=Warning  InternalRulePriority=Speed  RndMeth=Simplest  InputSameDT=on
  1-D Lookup Table3 : Lookup_n-D  NumberOfTableDimensions=1  BreakpointsForDimension1=breakpoints1  Table=Cmq  DiagnosticForOutOfRangeInput=Warning  InternalRulePriority=Speed  RndMeth=Simplest  InputSameDT=on
  Cm0 : Outport
  Cmde : Outport  Port=2
  de_deg : Outport  Port=3
  Cmq : Outport  Port=4
  wires:
  1-D Lookup Table/1 -> de_deg/1  "de_deg"
  1-D Lookup Table1/1 -> Cm0/1  "Cm0"
  Alpha (deg)/1 -> 1-D Lookup Table3/1, 1-D Lookup Table/1, 1-D Lookup Table2/1, 1-D Lookup Table1/1  "Alpha (deg)"
  1-D Lookup Table3/1 -> Cmq/1  "Cmq"
  1-D Lookup Table2/1 -> Cmde/1  "Cmde"

== system Simulation_wrapped_4/Manoeuvre Rig (simulation)/Manoeuvre rig simulation/Aerodynamics lookup1 ==
  Alpha (deg) : Inport
  1-D Lookup Table : Lookup_n-D  NumberOfTableDimensions=1  BreakpointsForDimension1=breakpoints1  Table=de  DiagnosticForOutOfRangeInput=Warning  InternalRulePriority=Speed  RndMeth=Simplest  InputSameDT=on
  1-D Lookup Table1 : Lookup_n-D  NumberOfTableDimensions=1  BreakpointsForDimension1=breakpoints1  Table=Cm0  DiagnosticForOutOfRangeInput=Warning  InternalRulePriority=Speed  RndMeth=Simplest  InputSameDT=on
  1-D Lookup Table2 : Lookup_n-D  NumberOfTableDimensions=1  BreakpointsForDimension1=breakpoints1  Table=Cmde  DiagnosticForOutOfRangeInput=Warning  InternalRulePriority=Speed  RndMeth=Simplest  InputSameDT=on
  1-D Lookup Table3 : Lookup_n-D  NumberOfTableDimensions=1  BreakpointsForDimension1=breakpoints1  Table=Cmq  DiagnosticForOutOfRangeInput=Warning  InternalRulePriority=Speed  RndMeth=Simplest  InputSameDT=on
  Cm0 : Outport
  Cmde : Outport  Port=2
  de_deg : Outport  Port=3
  Cmq : Outport  Port=4
  wires:
  1-D Lookup Table/1 -> de_deg/1  "de_deg"
  1-D Lookup Table1/1 -> Cm0/1  "Cm0"
  Alpha (deg)/1 -> 1-D Lookup Table3/1, 1-D Lookup Table/1, 1-D Lookup Table2/1, 1-D Lookup Table1/1  "Alpha (deg)"
  1-D Lookup Table3/1 -> Cmq/1  "Cmq"
  1-D Lookup Table2/1 -> Cmde/1  "Cmde"

== system Simulation_wrapped_4/Manoeuvre Rig (simulation)/Manoeuvre rig simulation/Compensator servo model1 ==
  Command : Inport
  Mot : Gain  Gain=K2_svo_cmp
  Saturation : Saturate  UpperLimit=max_rate_sat_cmp  LowerLimit=-max_rate_sat_cmp
  Sum : Sum  Inputs=|+-
  Sum1 : Sum  Inputs=|+-
  Svo : Gain  Gain=K1_svo_cmp
  kinematic : Subsystem
  Response : Outport
  wires:
  Sum/1 -> Svo/1
  Svo/1 -> Saturation/1
  Sum1/1 -> Mot/1
  Saturation/1 -> Sum1/1
  kinematic/1(de) -> Response/1, Sum/2
  Mot/1 -> kinematic/1(rate_dot)
  kinematic/2(de_dot) -> Sum1/2
  Command/1 -> Sum/1

== system Simulation_wrapped_4/Manoeuvre Rig (simulation)/Manoeuvre rig simulation/Compensator servo model2 ==
  Command : Inport
  Mot : Gain  Gain=K2_svo_cmp
  Saturation : Saturate  UpperLimit=max_rate_sat_cmp  LowerLimit=-max_rate_sat_cmp
  Sum : Sum  Inputs=|+-
  Sum1 : Sum  Inputs=|+-
  Svo : Gain  Gain=K1_svo_cmp
  kinematic : Subsystem
  Response : Outport
  wires:
  Command/1 -> Sum/1
  kinematic/2(de_dot) -> Sum1/2
  Mot/1 -> kinematic/1(rate_dot)
  kinematic/1(de) -> Sum/2, Response/1
  Saturation/1 -> Sum1/1
  Sum1/1 -> Mot/1
  Svo/1 -> Saturation/1
  Sum/1 -> Svo/1

== system Simulation_wrapped_4/Manoeuvre Rig (simulation)/Manoeuvre rig simulation/Compensator servo model3 ==
  Command : Inport
  Mot : Gain  Gain=K2_svo_cmp
  Saturation : Saturate  UpperLimit=max_rate_sat_cmp  LowerLimit=-max_rate_sat_cmp
  Sum : Sum  Inputs=|+-
  Sum1 : Sum  Inputs=|+-
  Svo : Gain  Gain=K1_svo_cmp
  kinematic : Subsystem
  Response : Outport
  wires:
  Sum/1 -> Svo/1
  Svo/1 -> Saturation/1
  Sum1/1 -> Mot/1
  Saturation/1 -> Sum1/1
  kinematic/1(de) -> Response/1, Sum/2
  Mot/1 -> kinematic/1(rate_dot)
  kinematic/2(de_dot) -> Sum1/2
  Command/1 -> Sum/1

== system Simulation_wrapped_4/Manoeuvre Rig (simulation)/Manoeuvre rig simulation/Compensator servo model4 ==
  Command : Inport
  Mot : Gain  Gain=K2_svo_cmp
  Saturation : Saturate  UpperLimit=max_rate_sat_cmp  LowerLimit=-max_rate_sat_cmp
  Sum : Sum  Inputs=|+-
  Sum1 : Sum  Inputs=|+-
  Svo : Gain  Gain=K1_svo_cmp
  kinematic : Subsystem
  Response : Outport
  wires:
  Command/1 -> Sum/1
  kinematic/2(de_dot) -> Sum1/2
  Mot/1 -> kinematic/1(rate_dot)
  kinematic/1(de) -> Sum/2, Response/1
  Saturation/1 -> Sum1/1
  Sum1/1 -> Mot/1
  Svo/1 -> Saturation/1
  Sum/1 -> Svo/1

== system Simulation_wrapped_4/Manoeuvre Rig (simulation)/Manoeuvre rig simulation/Extracting position vector 1 ==
  In1 : Inport
  MATLAB Function : MATLAB Function  TreatAsAtomicUnit=on
  Out1 : Outport
  wires:
  In1/1 -> MATLAB Function/1(u)
  MATLAB Function/1(y) -> Out1/1

== system Simulation_wrapped_4/Manoeuvre Rig (simulation)/Manoeuvre rig simulation/Extracting position vector 10 ==
  In1 : Inport
  MATLAB Function : MATLAB Function  TreatAsAtomicUnit=on
  Out1 : Outport
  wires:
  MATLAB Function/1(y) -> Out1/1
  In1/1 -> MATLAB Function/1(u)

== system Simulation_wrapped_4/Manoeuvre Rig (simulation)/Manoeuvre rig simulation/Extracting position vector 2 ==
  In1 : Inport
  MATLAB Function : MATLAB Function  TreatAsAtomicUnit=on
  Out1 : Outport
  wires:
  In1/1 -> MATLAB Function/1(u)
  MATLAB Function/1(y) -> Out1/1

== system Simulation_wrapped_4/Manoeuvre Rig (simulation)/Manoeuvre rig simulation/Extracting position vector 2  ==
  In1 : Inport
  MATLAB Function : MATLAB Function  TreatAsAtomicUnit=on
  Out1 : Outport
  wires:
  MATLAB Function/1(y) -> Out1/1
  In1/1 -> MATLAB Function/1(u)

== system Simulation_wrapped_4/Manoeuvre Rig (simulation)/Manoeuvre rig simulation/Extracting position vector 3 ==
  In1 : Inport
  MATLAB Function : MATLAB Function  TreatAsAtomicUnit=on
  Out1 : Outport
  wires:
  In1/1 -> MATLAB Function/1(u)
  MATLAB Function/1(y) -> Out1/1

== system Simulation_wrapped_4/Manoeuvre Rig (simulation)/Manoeuvre rig simulation/Extracting position vector 4 ==
  In1 : Inport
  MATLAB Function : MATLAB Function  TreatAsAtomicUnit=on
  Out1 : Outport
  wires:
  MATLAB Function/1(y) -> Out1/1
  In1/1 -> MATLAB Function/1(u)

== system Simulation_wrapped_4/Manoeuvre Rig (simulation)/Manoeuvre rig simulation/Extracting position vector 5 ==
  In1 : Inport
  MATLAB Function : MATLAB Function  TreatAsAtomicUnit=on
  Out1 : Outport
  wires:
  MATLAB Function/1(y) -> Out1/1
  In1/1 -> MATLAB Function/1(u)

== system Simulation_wrapped_4/Manoeuvre Rig (simulation)/Manoeuvre rig simulation/Extracting position vector 7 ==
  In1 : Inport
  MATLAB Function : MATLAB Function  TreatAsAtomicUnit=on
  Out1 : Outport
  wires:
  In1/1 -> MATLAB Function/1(u)
  MATLAB Function/1(y) -> Out1/1

== system Simulation_wrapped_4/Manoeuvre Rig (simulation)/Manoeuvre rig simulation/Extracting position vector 8 ==
  In1 : Inport
  MATLAB Function : MATLAB Function  TreatAsAtomicUnit=on
  Out1 : Outport
  wires:
  In1/1 -> MATLAB Function/1(u)
  MATLAB Function/1(y) -> Out1/1

== system Simulation_wrapped_4/Manoeuvre Rig (simulation)/Manoeuvre rig simulation/Hawk servo model ==
  note: Above saturation
      | represents voltage
      | saturation
  Command : Inport
  Mot : Gain  Gain=K2_svo_acm
  Saturation : Saturate  UpperLimit=max_rate_sat_acm  LowerLimit=-max_rate_sat_acm
  Sum : Sum  Inputs=|+-
  Sum1 : Sum  Inputs=|+-
  Svo : Gain  Gain=K1_svo_acm
  kinematic : Subsystem
  Response : Outport
  wires:
  Sum/1 -> Svo/1
  Svo/1 -> Saturation/1
  Sum1/1 -> Mot/1
  Saturation/1 -> Sum1/1
  kinematic/1(de) -> Response/1, Sum/2
  Mot/1 -> kinematic/1(rate_dot)
  kinematic/2(de_dot) -> Sum1/2
  Command/1 -> Sum/1
